simulink model "Fixed_SquadCopter_Closed_Loop_SMC"  (R2023a)
settings: Solver=ode4  StartTime=0.0  StopTime=20  FixedStep=0.01  RelTol=1e-3
undefined symbols (not defined in the file): sigbuilder_block
libraries: simulink_extras x23
settings Model: Creator=karee  LastModifiedBy=Nada Tamer
settings SolverCC: AlgebraicLoopSolver=TrustRegion
settings DataIOCC: ReturnWorkspaceOutputs=off
settings DebuggingCC: UnconnectedInputMsg=warning  UnconnectedOutputMsg=warning  UnconnectedLineMsg=warning  ArithmeticOperatorsInVariantConditions=warning
settings ModelReferenceCC: EnableRefExpFcnMdlSchedulingChecks=on
settings SFSimCC: SimUseLocalCustomCode=off  CustomCodeUndefinedFunction=UseInterfaceOnly
settings RTWCC: RTWUseLocalCustomCode=off

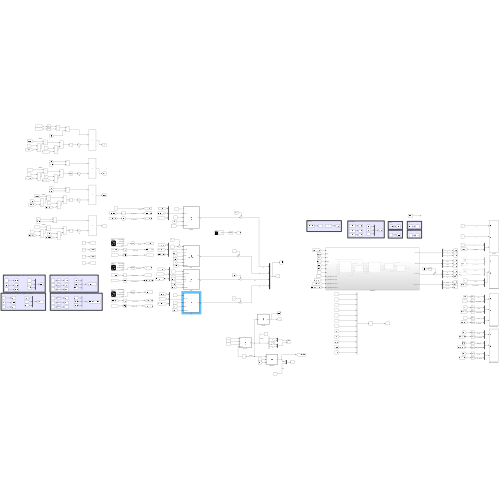
[thumbnail: Simulink's stored preview of the top-level diagram]
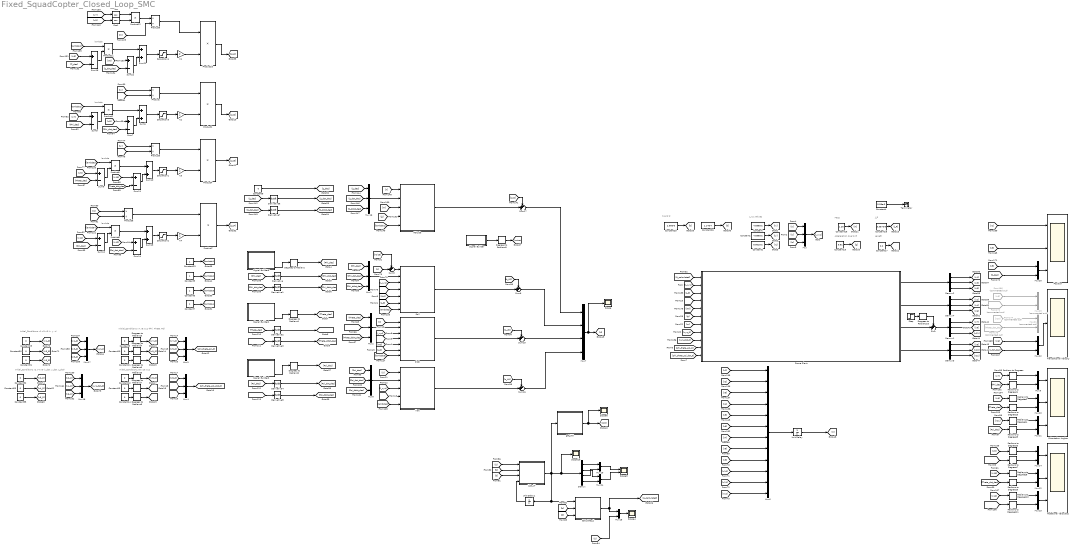
== system Fixed_SquadCopter_Closed_Loop_SMC ==
  note: b and d
  note: lambda
  note: Acceleration due to G
  note: I_xyz Values
  note: Mass
  note: Length
  note: J_R
  note: lambda
  note: lambda
  note: Initial_Conditions x7,x9,x11 (Phi, Theta, Psi)
  note: Initial_Conditions x8,x10,x12
  note: lambda
  note: Initial_Conditions x1,x3,x5 (x, y, z)
  note: Initial_Conditions x2,x4,x6 (x_dot, y_dot, z_dot)
  Attitude : MATLAB Function  TreatAsAtomicUnit=on
  Calculate_U : MATLAB Function  TreatAsAtomicUnit=on
  Constant : Constant  Value=4.856e-2
  Constant1 : Constant  Value=4.856e-2
  Constant{8..14,29..33,35} (13 alike) : Constant  Value=0
  Constant15 : Constant  Value=9.81
  Constant16 : Constant  Value=1.26
  Constant17 : Constant  Value=0.2
  Constant18 : Constant  Value=3.357e-5
  Constant2 : Constant  Value=8.801e-2
  Constant{5..7,23} (4 alike) : Constant
  Constant25 : Constant  Value=2.98e-6
  Constant26 : Constant  Value=1.14e-7
  Constant4 : Constant  Value=5.58e-3
  Cos : Trigonometry  Operator=cos
  Cos1 : Trigonometry  Operator=cos
  Degrees to Radians{,1..10} (11 alike) : simulink_extras/Transformations/Degrees to Radians
  Demux : Demux
  Demux{1..4} (4 alike) : Demux  Outputs=3
  Derivative{,1..7} (8 alike) : Derivative
  Drone Plant : Subsystem
  From166 : From  Commented=on  GotoTag=x8
  From172 : From  Commented=on  GotoTag=Phi_dot_des
  From173 : From  Commented=on  GotoTag=Theta_dot_des
  From174 : From  Commented=on  GotoTag=x10
  K{1..4} (4 alike) : Gain  Gain=2
  Mux{,1..4,8,16..18} (9 alike) : Mux  Inputs=3
  Mux{9..15,19..20,22,24} (11 alike) : Mux  Inputs=2
  Mux21 : Mux  Commented=on  Inputs=2
  Mux23 : Mux  Commented=on  Inputs=2
  Mux6 : Mux  Inputs=12
  Mux7 : Mux
  Orientation Angles : Scope  NumInputPorts=3
  Pitch : MATLAB Function  TreatAsAtomicUnit=on
  Position : Scope  NumInputPorts=3
  Product{,3,6,9} (4 alike) : Product  Inputs=*/
  Product{1..2,4..5,7..8,10..12} (9 alike) : Product  Inputs=**
  Radians to Degrees{,1..11} (12 alike) : simulink_extras/Transformations/Radians to Degrees
  Roll : MATLAB Function  TreatAsAtomicUnit=on
  Rotational Velocities : Scope  NumInputPorts=3
  Saturation{1..4} (4 alike) : Saturate  UpperLimit=1  LowerLimit=-1
  Scope{,4,6,10} (4 alike) : Scope
  Scope3 : Scope  NumInputPorts=2
  Signal Builder : Subsystem  Tag=STV Subsys  LoadFcn=sigbuilder_block('load');  StartFcn=sigbuilder_block('start');  StopFcn=sigbuilder_block('stop');  ClipboardFcn=sigbuilder_block('clipboard');  mask(Sigbuilder block){tuvar=[0:10]}
      mask help: Simulink:masks:SigbuilderBlock_MD
      mask init:
      | if ~strcmp(get_param(bdroot(gcbh),'SimulationStatus'),'stopped') tuvar = sigbuilder_block('maskInit'); end
      settings: CopyFcn=sigbuilder_block('copy');  DeleteFcn=sigbuilder_block('delete');  ModelCloseFcn=sigbuilder_block('modelClose');  PreSaveFcn=sigbuilder_block('preSave');  PauseFcn=sigbuilder_block('pause');  ContinueFcn=sigbuilder_block('continue');  NameChangeFcn=sigbuilder_block('namechange');  OpenFcn=sigbuilder_block('open',[437.25 153 550.5 359.25 ]);  CloseFcn=sigbuilder_block('close');
      mask Display: plot(0, 0, 100, 100,[2, 2, 32, 32, 2], [68, 8, 8, 68, 68],[32, 2], [38, 38], [32, 19, 2],[53, 60, 44], [32, 17, 17, 2],[16, 16, 31, 31]);txt = getActiveGroup(gcbh);text(2, 100, txt,'verticalAlignment', 'top');
  Signal Builder1 : Subsystem  Tag=STV Subsys  LoadFcn=sigbuilder_block('load');  StartFcn=sigbuilder_block('start');  StopFcn=sigbuilder_block('stop');  ClipboardFcn=sigbuilder_block('clipboard');  mask(Sigbuilder block){tuvar=[0:10]}
      mask help: Simulink:masks:SigbuilderBlock_MD
      mask init:
      | if ~strcmp(get_param(bdroot(gcbh),'SimulationStatus'),'stopped') tuvar = sigbuilder_block('maskInit'); end
      settings: CopyFcn=sigbuilder_block('copy');  DeleteFcn=sigbuilder_block('delete');  ModelCloseFcn=sigbuilder_block('modelClose');  PreSaveFcn=sigbuilder_block('preSave');  PauseFcn=sigbuilder_block('pause');  ContinueFcn=sigbuilder_block('continue');  NameChangeFcn=sigbuilder_block('namechange');  OpenFcn=sigbuilder_block('open',[0 30 1024.5 488.25 ]);  CloseFcn=sigbuilder_block('close');
      mask Display: plot(0, 0, 100, 100,[2, 2, 32, 32, 2], [68, 8, 8, 68, 68],[32, 2], [38, 38], [32, 19, 2],[53, 60, 44], [32, 17, 17, 2],[16, 16, 31, 31]);txt = getActiveGroup(gcbh);text(2, 100, txt,'verticalAlignment', 'top');
  Signal Builder2 : Subsystem  Tag=STV Subsys  LoadFcn=sigbuilder_block('load');  StartFcn=sigbuilder_block('start');  StopFcn=sigbuilder_block('stop');  ClipboardFcn=sigbuilder_block('clipboard');  mask(Sigbuilder block){tuvar=[0:10]}
      mask help: Simulink:masks:SigbuilderBlock_MD
      mask init:
      | if ~strcmp(get_param(bdroot(gcbh),'SimulationStatus'),'stopped') tuvar = sigbuilder_block('maskInit'); end
      settings: CopyFcn=sigbuilder_block('copy');  DeleteFcn=sigbuilder_block('delete');  ModelCloseFcn=sigbuilder_block('modelClose');  PreSaveFcn=sigbuilder_block('preSave');  PauseFcn=sigbuilder_block('pause');  ContinueFcn=sigbuilder_block('continue');  NameChangeFcn=sigbuilder_block('namechange');  OpenFcn=sigbuilder_block('open',[6 30 1012.5 447.75 ]);  CloseFcn=sigbuilder_block('close');
      mask Display: plot(0, 0, 100, 100,[2, 2, 32, 32, 2], [68, 8, 8, 68, 68],[32, 2], [38, 38], [32, 19, 2],[53, 60, 44], [32, 17, 17, 2],[16, 16, 31, 31]);txt = getActiveGroup(gcbh);text(2, 100, txt,'verticalAlignment', 'top');
  Signal Builder3 : Subsystem  Tag=STV Subsys  LoadFcn=sigbuilder_block('load');  StartFcn=sigbuilder_block('start');  StopFcn=sigbuilder_block('stop');  ClipboardFcn=sigbuilder_block('clipboard');  mask(Sigbuilder block){tuvar=[0:10]}
      mask help: Simulink:masks:SigbuilderBlock_MD
      mask init:
      | if ~strcmp(get_param(bdroot(gcbh),'SimulationStatus'),'stopped') tuvar = sigbuilder_block('maskInit'); end
      settings: CopyFcn=sigbuilder_block('copy');  DeleteFcn=sigbuilder_block('delete');  ModelCloseFcn=sigbuilder_block('modelClose');  PreSaveFcn=sigbuilder_block('preSave');  PauseFcn=sigbuilder_block('pause');  ContinueFcn=sigbuilder_block('continue');  NameChangeFcn=sigbuilder_block('namechange');  OpenFcn=sigbuilder_block('open',[6 30 1012.5 447.75 ]);  CloseFcn=sigbuilder_block('close');
      mask Display: plot(0, 0, 100, 100,[2, 2, 32, 32, 2], [68, 8, 8, 68, 68],[32, 2], [38, 38], [32, 19, 2],[53, 60, 44], [32, 17, 17, 2],[16, 16, 31, 31]);txt = getActiveGroup(gcbh);text(2, 100, txt,'verticalAlignment', 'top');
  Step : Step  Time=10  After=0  SampleTime=0
  Sum : Sum  Inputs=++|
  Sum{6,10,13,21} (4 alike) : Sum
  Sum{5,7,9,11..12,14,18,22} (8 alike) : Sum  Inputs=+-
  Sum{8,15..17} (4 alike) : Sum  Inputs=-+|
  Sum3 : Sum  Inputs=++|
  Terminator : Terminator
  Translational Velocity : Scope
  U_to_W : MATLAB Function  TreatAsAtomicUnit=on
  Unit Delay : UnitDelay  InitialCondition=[0;0;0;0;0;0;0;0;0;0;0;0]  SampleTime=0.01  HasFrameUpgradeWarning=on
  Unit Delay1 : UnitDelay  InitialCondition=[1018;1018;1018;1018]  SampleTime=0.01  HasFrameUpgradeWarning=on
  Yaw : MATLAB Function  TreatAsAtomicUnit=on
  get_Wd : MATLAB Function  TreatAsAtomicUnit=on
  wires:
  [Iz] -> Mux/3
  Constant1/1 -> [Iy]
  Constant2/1 -> [Iz]
  [Iy] -> Mux/2
  Constant/1 -> [Ix]
  Mux/1 -> [I_xyz]
  [Ix] -> Mux/1
  Constant15/1 -> [g]
  Constant16/1 -> [m]
  Constant17/1 -> [length]
  Constant18/1 -> [J_R]
  Constant25/1 -> [b]
  Constant26/1 -> [d]
  Demux1/3 -> [x11]  "psi"
  Demux1/2 -> [x9]  "theta"
  Demux3/1 -> [x8]  "phi_dot"
  Demux3/2 -> [x10]  "theta_dot"
  Demux3/3 -> [x12]  "psi_dot"
  [x8] -> Mux6/8
  [x10] -> Mux6/10
  [x12] -> Mux6/12
  Mux6/1 -> Unit Delay/1
  [I_xyz] -> Roll/3(I_xyz)
  [length] -> Roll/4(length)
  Mux7/1 -> Scope/1, [U]
  [U] -> U_to_W/1(U)
  [Wd] -> Roll/5(w_d)
  Mux1/1 -> Roll/2(PHI_des)
  Degrees to Radians/1 -> [Phi_des]  "Phi_des"
  [Phi_dot_des] -> Mux1/2
  [Phi_ddot_des] -> Mux1/3
  Mux2/1 -> Pitch/2(THETA_des)
  [X] -> Pitch/1(X)
  [I_xyz] -> Pitch/3(I_xyz)
  [length] -> Pitch/4(length)
  [Wd] -> Pitch/5(w_d)
  [I_xyz] -> Yaw/3(I_xyz)
  [X] -> Yaw/1(X)
  Mux8/1 -> Yaw/2(PSI_des)
  [length] -> Yaw/4(length)
  [x5] -> Mux6/5
  [x6] -> Mux6/6
  Unit Delay/1 -> [X]
  [J_R] -> Roll/6(J_r)
  [J_R] -> Pitch/6(J_r)
  [Ix] -> Product/1
  [length] -> Product/2
  Product/1 -> Product1/1
  [x7] -> Sum5/1
  [Phi_des] -> Mux1/1
  Derivative/1 -> [Phi_dot_des]  "Phi_dot_des"
  Derivative1/1 -> [Phi_ddot_des]  "Phi_ddot_des"
  [Phi_des] -> Sum5/2
  [lambda2] -> Product2/1
  Sum5/1 -> Product2/2
  Product2/1 -> Sum6/1
  [Phi_dot_des] -> Sum7/2
  [x8] -> Sum7/1
  Sum7/1 -> Sum6/2
  Sum6/1 -> Saturation3/1
  Saturation3/1 -> K2/1
  Roll/1(U2) -> Sum8/2  "U2"
  Sum8/1 -> Mux7/2  "U2"
  Derivative3/1 -> [Theta_ddot_des]  "Theta_ddot_des"
  Derivative2/1 -> [Theta_dot_des]  "Theta_dot_des"
  Degrees to Radians1/1 -> [Theta_des]  "Theta_des"
  [Theta_ddot_des] -> Mux2/3
  [Theta_des] -> Mux2/1
  [Theta_dot_des] -> Mux2/2
  Sum9/1 -> Product5/2
  [x10] -> Sum11/1
  Sum10/1 -> Saturation1/1
  Product3/1 -> Product4/1
  [length] -> Product3/2
  [x9] -> Sum9/1
  Sum11/1 -> Sum10/2
  [lambda3] -> Product5/1
  Saturation1/1 -> K3/1
  Product5/1 -> Sum10/1
  [Theta_des] -> Sum9/2
  [Theta_dot_des] -> Sum11/2
  [Iy] -> Product3/1
  Sum12/1 -> Product8/2
  [x12] -> Sum14/1
  Sum13/1 -> Saturation2/1
  Product6/1 -> Product7/1
  [length] -> Product6/2
  [x11] -> Sum12/1
  Sum14/1 -> Sum13/2
  [lambda4] -> Product8/1
  Saturation2/1 -> K4/1
  Product8/1 -> Sum13/1
  [Psi_des] -> Sum12/2
  [Psi_dot_des] -> Sum14/2
  [Iz] -> Product6/1
  Product1/1 -> [s_U2]
  Product4/1 -> [s_U3]
  Product7/1 -> [s_U4]
  Pitch/1(U3) -> Sum15/2  "U3"
  Yaw/1(U4) -> Sum16/2  "U4"
  Sum16/1 -> Mux7/4  "U4"
  Sum15/1 -> Mux7/3  "U3"
  [s_U2] -> Sum8/1
  [s_U3] -> Sum15/1
  [s_U4] -> Sum16/1
  Degrees to Radians2/1 -> [Psi_des]  "Psi_des"
  Derivative4/1 -> [Psi_dot_des]  "Psi_dot_des"
  Derivative5/1 -> [Psi_ddot_des]  "Psi_ddot_des"
  [Psi_des] -> Mux8/1
  [Psi_dot_des] -> Mux8/2
  [Psi_ddot_des] -> Mux8/3
  K4/1 -> Product7/2
  K3/1 -> Product4/2
  K2/1 -> Product1/2
  Mux9/1 -> Orientation Angles/1
  [x7] -> Radians to Degrees/1
  [Phi_des] -> Radians to Degrees1/1
  [Theta_des] -> Radians to Degrees3/1
  [x9] -> Radians to Degrees2/1
  Mux10/1 -> Orientation Angles/2
  Mux11/1 -> Orientation Angles/3
  [x11] -> Radians to Degrees4/1
  [Psi_des] -> Radians to Degrees5/1
  [Psi_dot_des] -> Radians to Degrees11/1
  [x12] -> Radians to Degrees10/1
  Mux13/1 -> Rotational Velocities/3
  Mux12/1 -> Rotational Velocities/2
  [x10] -> Radians to Degrees8/1
  [Theta_dot_des] -> Radians to Degrees9/1
  [Phi_dot_des] -> Radians to Degrees7/1
  [x8] -> Radians to Degrees6/1
  Mux14/1 -> Rotational Velocities/1
  Radians to Degrees/1 -> Mux9/1  "Phi"
  Radians to Degrees1/1 -> Mux9/2  "Phi_desired"
  Radians to Degrees2/1 -> Mux10/1  "Theta"
  Radians to Degrees3/1 -> Mux10/2  "Theta_desired"
  Radians to Degrees4/1 -> Mux11/1  "Psi"
  Radians to Degrees5/1 -> Mux11/2  "Psi_desired"
  Radians to Degrees7/1 -> Mux14/2  "Phi_dot_desired"
  Radians to Degrees6/1 -> Mux14/1  "Phi_dot"
  Radians to Degrees8/1 -> Mux12/1  "Theta_dot"
  Radians to Degrees9/1 -> Mux12/2  "Theta_dot_desired"
  Radians to Degrees10/1 -> Mux13/1  "Psi_dot"
  Radians to Degrees11/1 -> Mux13/2  "Psi_dot_desired"
  [Phi_des] -> Derivative/1
  [Phi_dot_des] -> Derivative1/1
  [Theta_dot_des] -> Derivative3/1
  [Theta_des] -> Derivative2/1
  [Psi_des] -> Derivative4/1
  [Theta_dot_des] -> Derivative5/1
  [d] -> U_to_W/3(d)
  [b] -> U_to_W/2(b)
  [b] -> Calculate_U/2(b)
  [d] -> Calculate_U/3(d)
  U_to_W/1(W) -> Scope10/1, Demux/1, get_Wd/1(W), Unit Delay1/1, Calculate_U/1(W)  "Omegas"
  Calculate_U/1(U) -> [U_calculated], Mux15/1  "Ucalc"
  [U] -> Mux15/2  "Uact"
  get_Wd/1(Wd) -> Scope6/1, [Wd]
  Constant5/1 -> [lambda2]
  Constant6/1 -> [lambda3]
  Constant7/1 -> [lambda4]
  [lambda2] -> Roll/7(lambda2)
  [lambda3] -> Pitch/7(lambda3)
  [lambda4] -> Yaw/5(lambda4)
  Constant14/1 -> Degrees to Radians8/1
  Degrees to Radians8/1 -> [x12_0]
  [x7_0] -> Mux3/1
  Degrees to Radians3/1 -> [x7_0]
  Degrees to Radians5/1 -> [x11_0]
  Mux3/1 -> [phi_theta_psi_0]
  Degrees to Radians4/1 -> [x9_0]
  [x9_0] -> Mux3/2
  [x12_0] -> Mux4/3
  Mux4/1 -> [phi_theta_psi_dot_0]
  Constant11/1 -> Degrees to Radians5/1
  Constant10/1 -> Degrees to Radians4/1
  [x10_0] -> Mux4/2
  [x8_0] -> Mux4/1
  Constant12/1 -> Degrees to Radians6/1
  Degrees to Radians7/1 -> [x10_0]
  Constant13/1 -> Degrees to Radians7/1
  Constant9/1 -> Degrees to Radians3/1
  Degrees to Radians6/1 -> [x8_0]
  [x11_0] -> Mux3/3
  [g] -> Attitude/4(g)
  Mux16/1 -> Attitude/2(Z_des)
  [lambda1] -> Attitude/5(lambda1)
  Constant8/1 -> [Z_des]  "Phi_des"
  [X] -> Attitude/1(X)
  Derivative6/1 -> [Z_dot_des]  "Phi_dot_des"
  [Z_des] -> Mux16/1
  [Z_dot_des] -> Derivative7/1
  Sum17/1 -> Mux7/1  "U1"
  [Z_dot_des] -> Mux16/2
  [s_U1] -> Sum17/1
  Derivative7/1 -> [Z_ddot_des]  "Phi_ddot_des"
  Attitude/1(U1) -> Sum17/2  "U1"
  [m] -> Attitude/3(m)
  [Z_des] -> Derivative6/1
  [Z_ddot_des] -> Mux16/3
  Product12/1 -> Product9/1
  Cos/1 -> Product12/1
  [m] -> Product9/2
  [x9] -> Cos1/1
  [x7] -> Cos/1
  [Z_des] -> Sum18/2
  Saturation4/1 -> K1/1
  [x6] -> Sum22/1
  [lambda1] -> Product11/1
  [Z_dot_des] -> Sum22/2
  Sum22/1 -> Sum21/2
  K1/1 -> Product10/2
  Product10/1 -> [s_U1]
  Sum18/1 -> Product11/2
  [x5] -> Sum18/1
  Product9/1 -> Product10/1
  Sum21/1 -> Saturation4/1
  Product11/1 -> Sum21/1
  Cos1/1 -> Product12/2
  [U_calculated] -> Drone Plant/1(u)
  Drone Plant/4("x8, x10, x12") -> Demux3/1
  [I_xyz] -> Drone Plant/2(I_xyz)
  [phi_theta_psi_dot_0] -> Drone Plant/11("Init_Conditions x8, x10, x12,")
  [xyz_dot_0] -> Drone Plant/9("Init_Conditions x2, x4, x6,")
  [J_R] -> Drone Plant/3(J_R)
  [xyz_0] -> Drone Plant/8("Init_Conditions x1, x3, x5")
  [phi_theta_psi_0] -> Drone Plant/10("Init_Conditions x7, x9, x11,")
  [g] -> Drone Plant/6(g)
  [length] -> Drone Plant/4(length)
  [m] -> Drone Plant/7(m)
  [Wd] -> Drone Plant/5(wd)
  Demux4/3 -> [x6]  "z_dot"
  Demux4/2 -> [x4]  "y_dot"
  Demux4/1 -> [x2]  "x_dot"
  Demux2/1 -> [x1]  "x"
  Demux2/2 -> [x3]  "y"
  Demux2/3 -> [x5]  "z"
  Drone Plant/2("x2, x4, x6") -> Demux4/1
  Drone Plant/1("x1, x3, x5") -> Demux2/1
  Constant33/1 -> [x4_0]
  [x5_0] -> Mux17/3
  Constant30/1 -> [x3_0]
  [x3_0] -> Mux17/2
  Mux17/1 -> [xyz_0]
  [x6_0] -> Mux18/3
  Constant35/1 -> [x6_0]
  [x4_0] -> Mux18/2
  [x1_0] -> Mux17/1
  Constant29/1 -> [x1_0]
  Constant31/1 -> [x5_0]
  [x2_0] -> Mux18/1
  Mux18/1 -> [xyz_dot_0]
  Constant32/1 -> [x2_0]
  [Z_dot_des] -> Mux22/2  "Z_dot_desired"
  [x6] -> Mux22/1  "Z_dot"
  From173/1 -> Mux21/2  "Theta_dot_desired"
  From174/1 -> Mux21/1  "Theta_dot"
  From166/1 -> Mux23/1  "Phi_dot"
  From172/1 -> Mux23/2  "Phi_dot_desired"
  [Z_des] -> Mux20/2  "Z_desired"
  [x5] -> Mux20/1  "Z"
  [x3] -> Position/2  "Y"
  [x1] -> Position/1  "X"
  Mux22/1 -> Translational Velocity/1
  Constant23/1 -> [lambda1]
  Demux1/1 -> [x7]  "phi"
  Mux20/1 -> Position/3
  [x4] -> Mux6/4
  [x3] -> Mux6/3
  [x2] -> Mux6/2
  [x1] -> Mux6/1
  Demux/1 -> Mux19/1  "w1"
  Mux19/1 -> Scope3/1
  Demux/3 -> Mux19/2  "w3"
  Mux24/1 -> Scope3/2
  Demux/2 -> Mux24/1  "w2"
  Demux/4 -> Mux24/2  "w4"
  Constant4/1 -> Terminator/1
  Mux15/1 -> Scope4/1
  Unit Delay1/1 -> U_to_W/4(W_old)
  Signal Builder1/4(Zero) -> Degrees to Radians1/1
  Signal Builder/1(Noise) -> Degrees to Radians9/1
  Degrees to Radians9/1 -> [noise]
  [x7] -> Mux6/7
  [x9] -> Mux6/9
  [x11] -> Mux6/11
  [noise] -> Sum3/1
  Sum3/1 -> Roll/1(X)
  [X] -> Sum3/2
  Sum/1 -> Demux1/1
  Drone Plant/3("x7, x9, x11") -> Sum/2
  Step/1 -> Degrees to Radians10/1
  Signal Builder3/4(Zero) -> Degrees to Radians/1
  Degrees to Radians10/1 -> Sum/1
  Signal Builder2/4(Zero) -> Degrees to Radians2/1

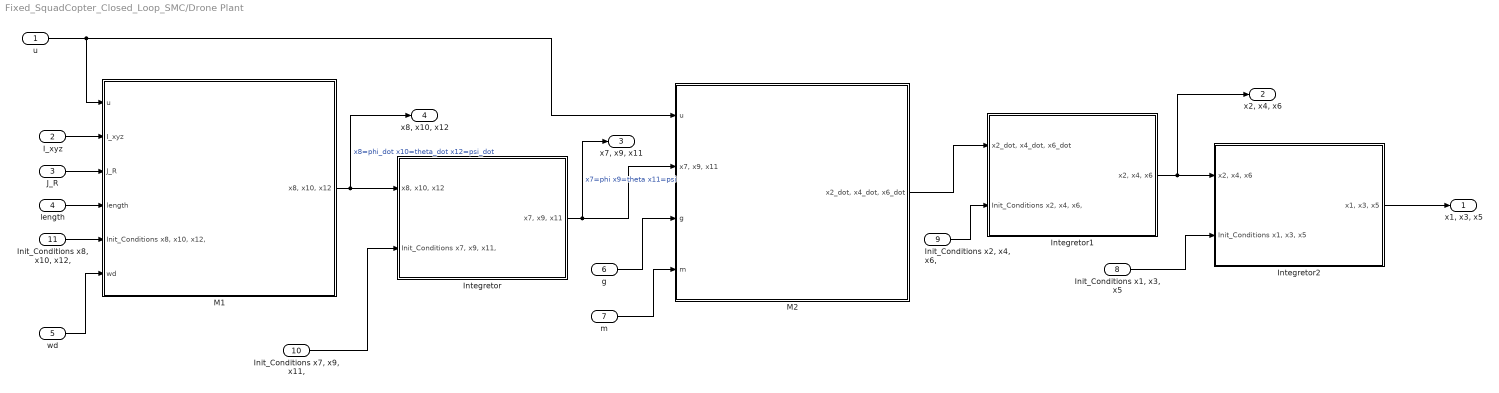
== system Fixed_SquadCopter_Closed_Loop_SMC/Drone Plant ==
  u : Inport
  I_xyz : Inport  Port=2
  J_R : Inport  Port=3
  length : Inport  Port=4
  wd : Inport  Port=5
  g : Inport  Port=6
  m : Inport  Port=7
  "Init_Conditions x1, x3, x5" : Inport  Port=8
  "Init_Conditions x2, x4, x6," : Inport  Port=9
  "Init_Conditions x7, x9, x11," : Inport  Port=10
  "Init_Conditions x8, x10, x12," : Inport  Port=11
  Integretor : Subsystem
  Integretor1 : Subsystem
  Integretor2 : Subsystem
  M1 : Subsystem
  M2 : Subsystem
  "x1, x3, x5" : Outport  VectorParamsAs1DForOutWhenUnconnected=off
  "x2, x4, x6" : Outport  Port=2  VectorParamsAs1DForOutWhenUnconnected=off
  "x7, x9, x11" : Outport  Port=3  VectorParamsAs1DForOutWhenUnconnected=off
  "x8, x10, x12" : Outport  Port=4  VectorParamsAs1DForOutWhenUnconnected=off
  wires:
  Integretor2/1("x1, x3, x5") -> "x1, x3, x5"/1
  Integretor1/1("x2, x4, x6") -> "x2, x4, x6"/1, Integretor2/1("x2, x4, x6")
  Integretor/1("x7, x9, x11") -> "x7, x9, x11"/1, M2/2("x7, x9, x11")  "x7=phi x9=theta x11=psi"
  u/1 -> M1/1(u), M2/1(u)
  m/1 -> M2/4(m)
  M1/1("x8, x10, x12") -> "x8, x10, x12"/1, Integretor/1("x8, x10, x12")  "x8=phi_dot x10=theta_dot x12=psi_dot"
  "Init_Conditions x7, x9, x11,"/1 -> Integretor/2("Init_Conditions x7, x9, x11,")
  g/1 -> M2/3(g)
  "Init_Conditions x2, x4, x6,"/1 -> Integretor1/2("Init_Conditions x2, x4, x6,")
  "Init_Conditions x1, x3, x5"/1 -> Integretor2/2("Init_Conditions x1, x3, x5")
  "Init_Conditions x8, x10, x12,"/1 -> M1/5("Init_Conditions x8, x10, x12,")
  length/1 -> M1/4(length)
  M2/1("x2_dot, x4_dot, x6_dot") -> Integretor1/1("x2_dot, x4_dot, x6_dot")
  wd/1 -> M1/6(wd)
  J_R/1 -> M1/3(J_R)
  I_xyz/1 -> M1/2(I_xyz)

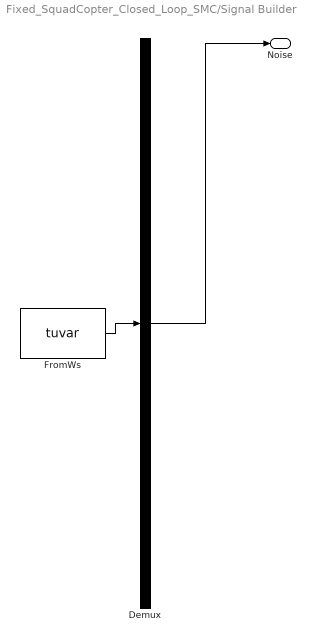
== system Fixed_SquadCopter_Closed_Loop_SMC/Signal Builder ==
  Demux : Demux  Tag=STV Demux  Outputs=1
      settings: DisplayOption=none
  FromWs : FromWorkspace  Tag=STV FromWs  VariableName=tuvar
      SigBuilderData=|
      | common.afterFinalStr = 'Extrapolate'
      | common.sampleTime = 0
      | dataSet.timeRange = [0 20]
      | dataSet.name = 'Group 1'
      | sbobj.Groups.Name = 'Group 1'
      | sbobj.Groups.Signals.Name = 'Noise'
      | sbobj.Groups.Signals.XData = [0 1 2 3 4 5 6 7 8 9 10 11 12 13 14 15 16 17 18 19 20]
      | sbobj.Groups.Signals.YData = [0.942376933302 0.0937254906669 -1.12231172153 0.306157818568 -1.17233486755 -0.960966563538 -0.653735016358 -1.229393649 -0.270965129963 -0.899950067343 -0.285686137602 -0.462421544354 -0.40978521474 -0.503538984132 1.23329711264 0.610305217574 0.0590721550527 -1.46694673043 -1.6258032664 -1.96475241539 2.60519575087]
      | sbobj.Groups.TimeRange = [0 20]
  Noise : Outport  Tag=STV Outport  VectorParamsAs1DForOutWhenUnconnected=off
  wires:
  Demux/1 -> Noise/1
  FromWs/1 -> Demux/1

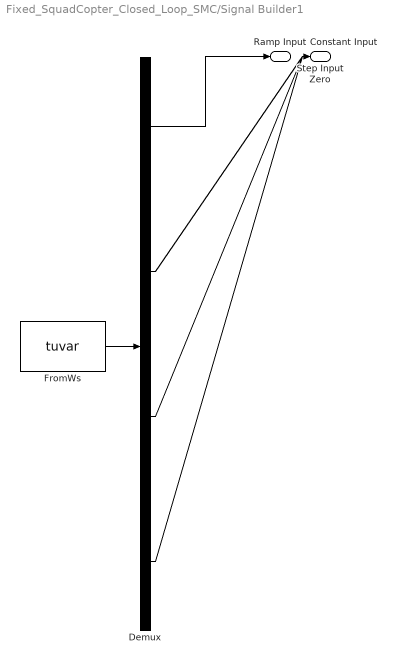
== system Fixed_SquadCopter_Closed_Loop_SMC/Signal Builder1 ==
  Demux : Demux  Tag=STV Demux
      settings: DisplayOption=none
  FromWs : FromWorkspace  Tag=STV FromWs  VariableName=tuvar
      SigBuilderData=|
      | common.afterFinalStr = 'Extrapolate'
      | common.sampleTime = 0
      | dataSet.timeRange = [0 20]
      | dataSet.name = 'Group 1'
      | sbobj.Groups.Name = 'Group 1'
      | sbobj.Groups.Signals(1).Name = 'Ramp Input'
      | sbobj.Groups.Signals(1).XData = [0 20]
      | sbobj.Groups.Signals(1).YData = [0 15]
      | sbobj.Groups.Signals(2).Name = 'Step Input'
      | sbobj.Groups.Signals(2).XData = [0 5 5 10 10 15 15 20]
      | sbobj.Groups.Signals(2).YData = [0 0 15 15 10 10 0 0]
      | sbobj.Groups.Signals(3).Name = 'Constant Input'
      | sbobj.Groups.Signals(3).XData = [0 20]
      | sbobj.Groups.Signals(3).YData = [10 10]
      | sbobj.Groups.Signals(4).Name = 'Zero'
      | sbobj.Groups.Signals(4).XData = [0 20]
      | sbobj.Groups.Signals(4).YData = [0 0]
      | sbobj.Groups.TimeRange = [0 20]
  Ramp Input : Outport  Tag=STV Outport  VectorParamsAs1DForOutWhenUnconnected=off
  Step Input : Outport  Tag=STV Outport  Port=2  VectorParamsAs1DForOutWhenUnconnected=off
  Constant Input : Outport  Tag=STV Outport  Port=3  VectorParamsAs1DForOutWhenUnconnected=off
  Zero : Outport  Tag=STV Outport  Port=4  VectorParamsAs1DForOutWhenUnconnected=off
  wires:
  Demux/3 -> Constant Input/1
  Demux/2 -> Step Input/1
  FromWs/1 -> Demux/1
  Demux/1 -> Ramp Input/1
  Demux/4 -> Zero/1

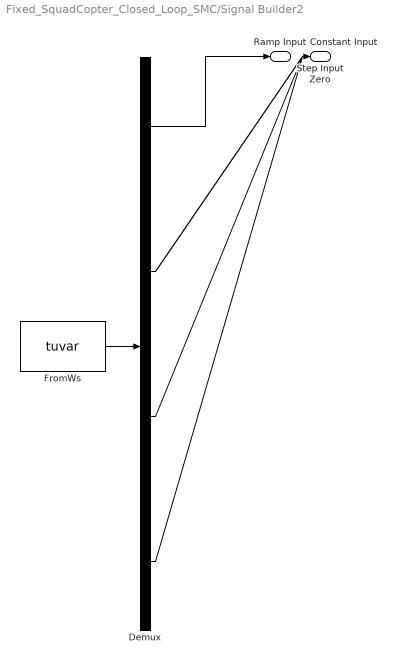
== system Fixed_SquadCopter_Closed_Loop_SMC/Signal Builder2 ==
  Demux : Demux  Tag=STV Demux
      settings: DisplayOption=none
  FromWs : FromWorkspace  Tag=STV FromWs  VariableName=tuvar
      SigBuilderData=|
      | common.afterFinalStr = 'Extrapolate'
      | common.sampleTime = 0
      | dataSet.timeRange = [0 20]
      | dataSet.name = 'Group 1'
      | sbobj.Groups.Name = 'Group 1'
      | sbobj.Groups.Signals(1).Name = 'Ramp Input'
      | sbobj.Groups.Signals(1).XData = [0 20]
      | sbobj.Groups.Signals(1).YData = [0 360]
      | sbobj.Groups.Signals(2).Name = 'Step Input'
      | sbobj.Groups.Signals(2).XData = [0 5 5 10 10 15 15 20]
      | sbobj.Groups.Signals(2).YData = [0 0 90 90 45 45 0 0]
      | sbobj.Groups.Signals(3).Name = 'Constant Input'
      | sbobj.Groups.Signals(3).XData = [0 20]
      | sbobj.Groups.Signals(3).YData = [180 180]
      | sbobj.Groups.Signals(4).Name = 'Zero'
      | sbobj.Groups.Signals(4).XData = [0 20]
      | sbobj.Groups.Signals(4).YData = [0 0]
      | sbobj.Groups.TimeRange = [0 20]
  Ramp Input : Outport  Tag=STV Outport  VectorParamsAs1DForOutWhenUnconnected=off
  Step Input : Outport  Tag=STV Outport  Port=2  VectorParamsAs1DForOutWhenUnconnected=off
  Constant Input : Outport  Tag=STV Outport  Port=3  VectorParamsAs1DForOutWhenUnconnected=off
  Zero : Outport  Tag=STV Outport  Port=4  VectorParamsAs1DForOutWhenUnconnected=off
  wires:
  Demux/1 -> Ramp Input/1
  FromWs/1 -> Demux/1
  Demux/2 -> Step Input/1
  Demux/3 -> Constant Input/1
  Demux/4 -> Zero/1

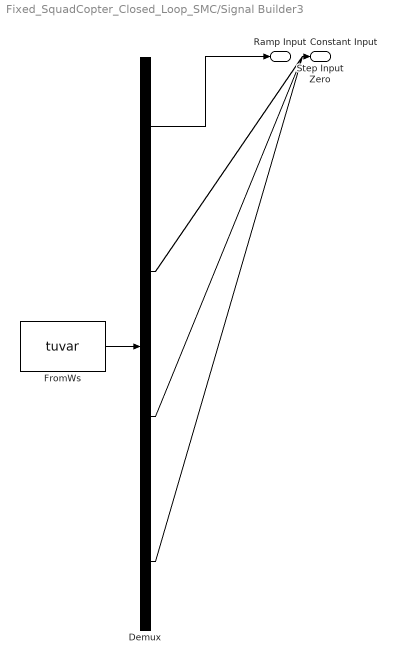
== system Fixed_SquadCopter_Closed_Loop_SMC/Signal Builder3 ==
  Demux : Demux  Tag=STV Demux
      settings: DisplayOption=none
  FromWs : FromWorkspace  Tag=STV FromWs  VariableName=tuvar
      SigBuilderData=|
      | common.afterFinalStr = 'Extrapolate'
      | common.sampleTime = 0
      | dataSet.timeRange = [0 20]
      | dataSet.name = 'Group 1'
      | sbobj.Groups.Name = 'Group 1'
      | sbobj.Groups.Signals(1).Name = 'Ramp Input'
      | sbobj.Groups.Signals(1).XData = [0 20]
      | sbobj.Groups.Signals(1).YData = [0 20]
      | sbobj.Groups.Signals(2).Name = 'Step Input'
      | sbobj.Groups.Signals(2).XData = [0 5 5 10 10 15 15 20]
      | sbobj.Groups.Signals(2).YData = [0 0 25 25 10 10 0 0]
      | sbobj.Groups.Signals(3).Name = 'Constant Input'
      | sbobj.Groups.Signals(3).XData = [0 20]
      | sbobj.Groups.Signals(3).YData = [20 20]
      | sbobj.Groups.Signals(4).Name = 'Zero'
      | sbobj.Groups.Signals(4).XData = [0 20]
      | sbobj.Groups.Signals(4).YData = [0 0]
      | sbobj.Groups.TimeRange = [0 20]
  Ramp Input : Outport  Tag=STV Outport  VectorParamsAs1DForOutWhenUnconnected=off
  Step Input : Outport  Tag=STV Outport  Port=2  VectorParamsAs1DForOutWhenUnconnected=off
  Constant Input : Outport  Tag=STV Outport  Port=3  VectorParamsAs1DForOutWhenUnconnected=off
  Zero : Outport  Tag=STV Outport  Port=4  VectorParamsAs1DForOutWhenUnconnected=off
  wires:
  Demux/4 -> Zero/1
  Demux/3 -> Constant Input/1
  Demux/2 -> Step Input/1
  FromWs/1 -> Demux/1
  Demux/1 -> Ramp Input/1

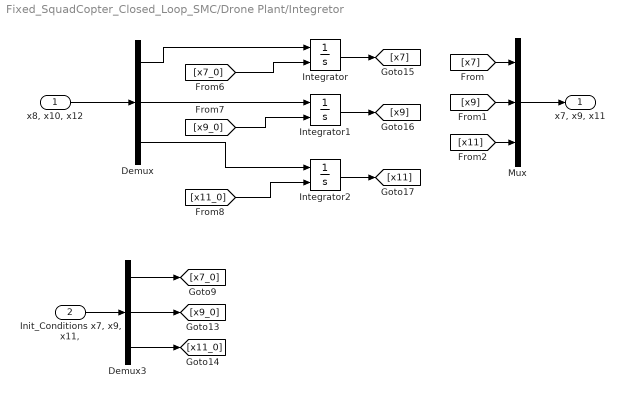
== system Fixed_SquadCopter_Closed_Loop_SMC/Drone Plant/Integretor ==
  "x8, x10, x12" : Inport
  "Init_Conditions x7, x9, x11," : Inport  Port=2
  Demux : Demux  Outputs=3
  Demux3 : Demux  Outputs=3
  Integrator : Integrator  InitialConditionSource=external
  Integrator1 : Integrator  InitialConditionSource=external
  Integrator2 : Integrator  InitialConditionSource=external
  Mux : Mux  Inputs=3
  "x7, x9, x11" : Outport  VectorParamsAs1DForOutWhenUnconnected=off
  wires:
  [x7] -> Mux/1
  [x11] -> Mux/3
  Demux3/3 -> [x11_0]
  Integrator2/1 -> [x11]
  [x11_0] -> Integrator2/2
  [x9] -> Mux/2
  "Init_Conditions x7, x9, x11,"/1 -> Demux3/1
  [x7_0] -> Integrator/2
  Mux/1 -> "x7, x9, x11"/1
  [x9_0] -> Integrator1/2
  Integrator/1 -> [x7]
  Demux/1 -> Integrator/1
  Integrator1/1 -> [x9]
  "x8, x10, x12"/1 -> Demux/1
  Demux/2 -> Integrator1/1
  Demux3/2 -> [x9_0]
  Demux3/1 -> [x7_0]
  Demux/3 -> Integrator2/1

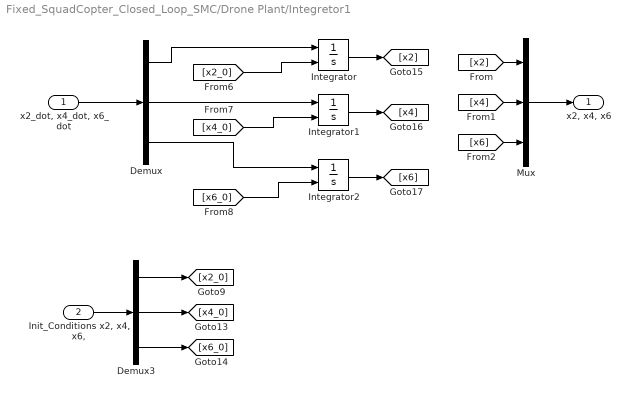
== system Fixed_SquadCopter_Closed_Loop_SMC/Drone Plant/Integretor1 ==
  "x2_dot, x4_dot, x6_dot" : Inport
  "Init_Conditions x2, x4, x6," : Inport  Port=2
  Demux : Demux  Outputs=3
  Demux3 : Demux  Outputs=3
  Integrator : Integrator  InitialConditionSource=external
  Integrator1 : Integrator  InitialConditionSource=external
  Integrator2 : Integrator  InitialConditionSource=external
  Mux : Mux  Inputs=3
  "x2, x4, x6" : Outport  VectorParamsAs1DForOutWhenUnconnected=off
  wires:
  Demux/3 -> Integrator2/1
  Demux3/1 -> [x2_0]
  Demux3/2 -> [x4_0]
  Demux/2 -> Integrator1/1
  "x2_dot, x4_dot, x6_dot"/1 -> Demux/1
  Integrator1/1 -> [x4]
  Demux/1 -> Integrator/1
  Integrator/1 -> [x2]
  [x4_0] -> Integrator1/2
  Mux/1 -> "x2, x4, x6"/1
  [x2_0] -> Integrator/2
  "Init_Conditions x2, x4, x6,"/1 -> Demux3/1
  [x4] -> Mux/2
  [x6_0] -> Integrator2/2
  Integrator2/1 -> [x6]
  Demux3/3 -> [x6_0]
  [x6] -> Mux/3
  [x2] -> Mux/1

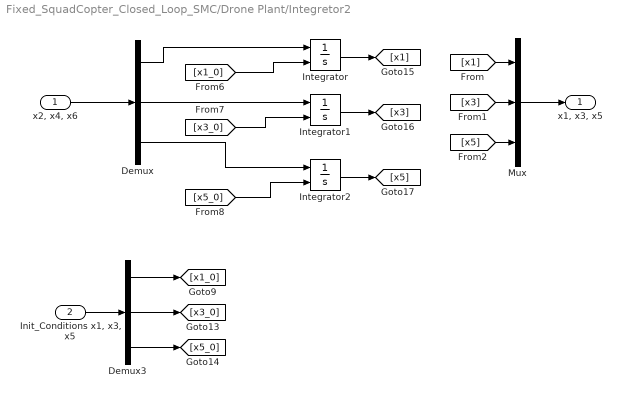
== system Fixed_SquadCopter_Closed_Loop_SMC/Drone Plant/Integretor2 ==
  "x2, x4, x6" : Inport
  "Init_Conditions x1, x3, x5" : Inport  Port=2
  Demux : Demux  Outputs=3
  Demux3 : Demux  Outputs=3
  Integrator : Integrator  InitialConditionSource=external
  Integrator1 : Integrator  InitialConditionSource=external
  Integrator2 : Integrator  InitialConditionSource=external
  Mux : Mux  Inputs=3
  "x1, x3, x5" : Outport  VectorParamsAs1DForOutWhenUnconnected=off
  wires:
  [x1] -> Mux/1
  [x5] -> Mux/3
  Demux3/3 -> [x5_0]
  Integrator2/1 -> [x5]
  [x5_0] -> Integrator2/2
  [x3] -> Mux/2
  "Init_Conditions x1, x3, x5"/1 -> Demux3/1
  [x1_0] -> Integrator/2
  Mux/1 -> "x1, x3, x5"/1
  [x3_0] -> Integrator1/2
  Integrator/1 -> [x1]
  Demux/1 -> Integrator/1
  Integrator1/1 -> [x3]
  "x2, x4, x6"/1 -> Demux/1
  Demux/2 -> Integrator1/1
  Demux3/2 -> [x3_0]
  Demux3/1 -> [x1_0]
  Demux/3 -> Integrator2/1

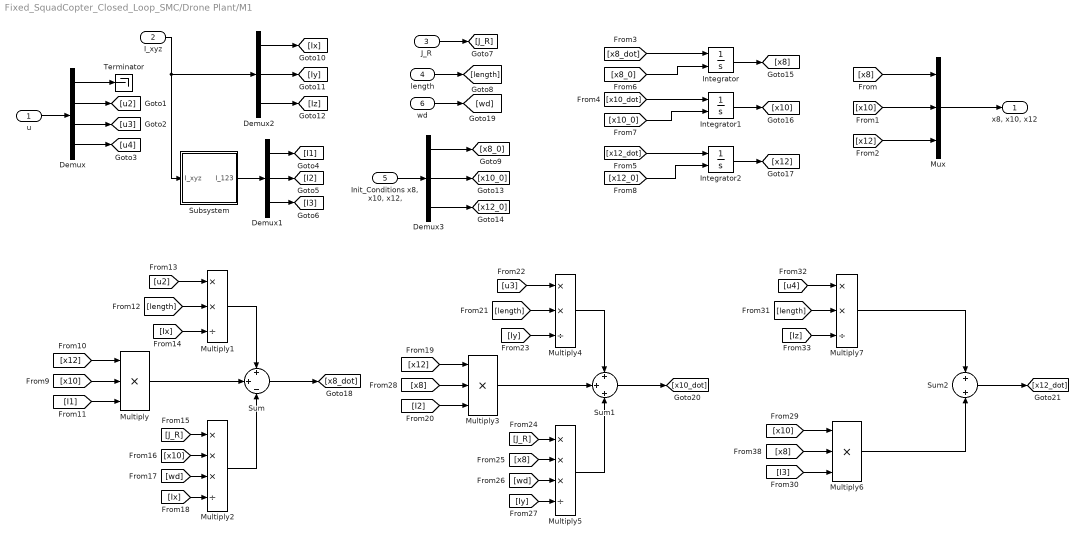
== system Fixed_SquadCopter_Closed_Loop_SMC/Drone Plant/M1 ==
  u : Inport
  I_xyz : Inport  Port=2
  J_R : Inport  Port=3
  length : Inport  Port=4
  "Init_Conditions x8, x10, x12," : Inport  Port=5
  wd : Inport  Port=6
  Demux : Demux
  Demux1 : Demux  Outputs=3
  Demux2 : Demux  Outputs=3
  Demux3 : Demux  Outputs=3
  Integrator : Integrator  InitialConditionSource=external
  Integrator1 : Integrator  InitialConditionSource=external
  Integrator2 : Integrator  InitialConditionSource=external
  Multiply : Product  Inputs=3
  Multiply1 : Product  Inputs=**/
  Multiply2 : Product  Inputs=***/
  Multiply3 : Product  Inputs=3
  Multiply4 : Product  Inputs=**/
  Multiply5 : Product  Inputs=***/
  Multiply6 : Product  Inputs=3
  Multiply7 : Product  Inputs=**/
  Mux : Mux  Inputs=3
  Subsystem : Subsystem
  Sum : Sum  Inputs=+|+|-
  Sum1 : Sum  Inputs=+|+|+
  Sum2 : Sum  Inputs=+|+
  Terminator : Terminator
  "x8, x10, x12" : Outport  VectorParamsAs1DForOutWhenUnconnected=off
  wires:
  u/1 -> Demux/1
  Demux/1 -> Terminator/1
  Demux/2 -> [u2]
  Demux/3 -> [u3]
  Demux/4 -> [u4]
  Demux2/2 -> [Iy]
  Demux2/3 -> [Iz]
  Demux2/1 -> [Ix]
  I_xyz/1 -> Demux2/1, Subsystem/1(I_xyz)
  Subsystem/1(I_123) -> Demux1/1
  Demux1/1 -> [I1]
  Demux1/2 -> [I2]
  Demux1/3 -> [I3]
  J_R/1 -> [J_R]
  length/1 -> [length]
  "Init_Conditions x8, x10, x12,"/1 -> Demux3/1
  Demux3/1 -> [x8_0]
  Demux3/3 -> [x12_0]
  Demux3/2 -> [x10_0]
  [x10] -> Mux/2
  [x8] -> Mux/1
  [x12] -> Mux/3
  Mux/1 -> "x8, x10, x12"/1
  [x12_dot] -> Integrator2/1
  [x8_dot] -> Integrator/1
  [x10_dot] -> Integrator1/1
  [x8_0] -> Integrator/2
  [x10_0] -> Integrator1/2
  [x12_0] -> Integrator2/2
  Integrator/1 -> [x8]
  Integrator1/1 -> [x10]
  Integrator2/1 -> [x12]
  Sum/1 -> [x8_dot]
  Multiply/1 -> Sum/2
  [x12] -> Multiply/1
  [x10] -> Multiply/2
  [I1] -> Multiply/3
  wd/1 -> [wd]
  [length] -> Multiply1/2
  [u2] -> Multiply1/1
  [Ix] -> Multiply1/3
  Multiply1/1 -> Sum/1
  [J_R] -> Multiply2/1
  [x10] -> Multiply2/2
  [wd] -> Multiply2/3
  [Ix] -> Multiply2/4
  Multiply2/1 -> Sum/3
  Multiply5/1 -> Sum1/3
  [Iy] -> Multiply5/4
  [wd] -> Multiply5/3
  [x8] -> Multiply5/2
  [J_R] -> Multiply5/1
  Multiply4/1 -> Sum1/1
  [Iy] -> Multiply4/3
  [u3] -> Multiply4/1
  [length] -> Multiply4/2
  [I2] -> Multiply3/3
  [x8] -> Multiply3/2
  [x12] -> Multiply3/1
  Multiply3/1 -> Sum1/2
  Sum1/1 -> [x10_dot]
  Sum2/1 -> [x12_dot]
  Multiply6/1 -> Sum2/2
  [x10] -> Multiply6/1
  [x8] -> Multiply6/2
  [I3] -> Multiply6/3
  [length] -> Multiply7/2
  [u4] -> Multiply7/1
  [Iz] -> Multiply7/3
  Multiply7/1 -> Sum2/1

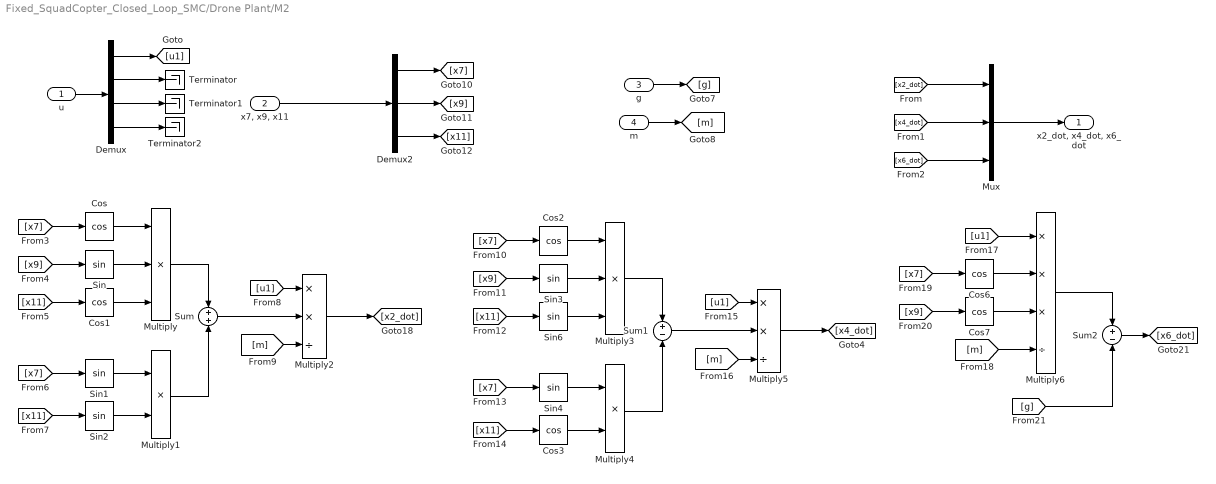
== system Fixed_SquadCopter_Closed_Loop_SMC/Drone Plant/M2 ==
  u : Inport
  "x7, x9, x11" : Inport  Port=2
  g : Inport  Port=3
  m : Inport  Port=4
  Cos{,1..3,6..7} (6 alike) : Trigonometry  Operator=cos
  Demux : Demux
  Demux2 : Demux  Outputs=3
  Multiply : Product  Inputs=3
  Multiply1 : Product
  Multiply2 : Product  Inputs=**/
  Multiply3 : Product  Inputs=3
  Multiply4 : Product
  Multiply5 : Product  Inputs=**/
  Multiply6 : Product  Inputs=***/
  Mux : Mux  Inputs=3
  Sin{,1..4,6} (6 alike) : Trigonometry
  Sum : Sum  Inputs=+|+
  Sum1 : Sum  Inputs=+|-
  Sum2 : Sum  Inputs=+|-
  Terminator : Terminator
  Terminator1 : Terminator
  Terminator2 : Terminator
  "x2_dot, x4_dot, x6_dot" : Outport  VectorParamsAs1DForOutWhenUnconnected=off
  wires:
  Mux/1 -> "x2_dot, x4_dot, x6_dot"/1
  [x6_dot] -> Mux/3
  [x2_dot] -> Mux/1
  [x4_dot] -> Mux/2
  m/1 -> [m]
  g/1 -> [g]
  Demux/4 -> Terminator2/1
  Demux/3 -> Terminator1/1
  Demux/2 -> Terminator/1
  Demux/1 -> [u1]
  u/1 -> Demux/1
  "x7, x9, x11"/1 -> Demux2/1
  Demux2/1 -> [x7]
  Demux2/3 -> [x11]
  Demux2/2 -> [x9]
  Multiply/1 -> Sum/1
  Multiply1/1 -> Sum/2
  Sum/1 -> Multiply2/2
  Multiply2/1 -> [x2_dot]
  Sin/1 -> Multiply/2
  Cos/1 -> Multiply/1
  Cos1/1 -> Multiply/3
  [x7] -> Cos/1
  [x9] -> Sin/1
  [x11] -> Cos1/1
  Sin1/1 -> Multiply1/1
  Sin2/1 -> Multiply1/2
  [x7] -> Sin1/1
  [x11] -> Sin2/1
  [u1] -> Multiply2/1
  [m] -> Multiply2/3
  [m] -> Multiply5/3
  [u1] -> Multiply5/1
  [x11] -> Cos3/1
  [x7] -> Sin4/1
  Cos3/1 -> Multiply4/2
  Sin4/1 -> Multiply4/1
  [x11] -> Sin6/1
  [x9] -> Sin3/1
  [x7] -> Cos2/1
  Sin6/1 -> Multiply3/3
  Cos2/1 -> Multiply3/1
  Sin3/1 -> Multiply3/2
  Multiply5/1 -> [x4_dot]
  Sum1/1 -> Multiply5/2
  Multiply4/1 -> Sum1/2
  Multiply3/1 -> Sum1/1
  [x9] -> Cos7/1
  Cos7/1 -> Multiply6/3
  Cos6/1 -> Multiply6/2
  [x7] -> Cos6/1
  [u1] -> Multiply6/1
  [m] -> Multiply6/4
  Multiply6/1 -> Sum2/1
  [g] -> Sum2/2
  Sum2/1 -> [x6_dot]

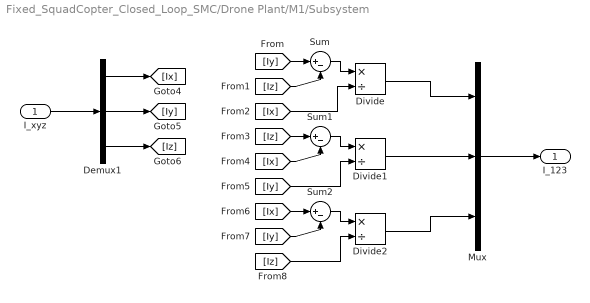
== system Fixed_SquadCopter_Closed_Loop_SMC/Drone Plant/M1/Subsystem ==
  I_xyz : Inport
  Demux1 : Demux  Outputs=3
  Divide : Product  Inputs=*/
  Divide1 : Product  Inputs=*/
  Divide2 : Product  Inputs=*/
  Mux : Mux  Inputs=3
  Sum : Sum  Inputs=|+-
  Sum1 : Sum  Inputs=|+-
  Sum2 : Sum  Inputs=|+-
  I_123 : Outport  VectorParamsAs1DForOutWhenUnconnected=off
  wires:
  [Iy] -> Sum2/2
  Divide2/1 -> Mux/3
  [Iy] -> Sum/1
  Sum/1 -> Divide/1
  I_xyz/1 -> Demux1/1
  Sum2/1 -> Divide2/1
  [Ix] -> Sum2/1
  [Iz] -> Divide2/2
  Demux1/3 -> [Iz]
  [Ix] -> Sum1/2
  Demux1/1 -> [Ix]
  [Ix] -> Divide/2
  [Iz] -> Sum/2
  Divide/1 -> Mux/1
  Sum1/1 -> Divide1/1
  Divide1/1 -> Mux/2
  [Iz] -> Sum1/1
  [Iy] -> Divide1/2
  Demux1/2 -> [Iy]
  Mux/1 -> I_123/1

== matlab function Fixed_SquadCopter_Closed_Loop_SMC/Roll ==
  data: X input; U2 output; PHI_des input; I_xyz input; length input; w_d input; J_r input; lambda2 input
function U2 = Roll_Control(X,PHI_des,I_xyz,length,w_d,J_r,lambda2)
lambda=lambda2;
% k1=2;
% k2=2;
k=2;

Ix=I_xyz(1);
Iy=I_xyz(2);
Iz=I_xyz(3);

b1=length/Ix;

a1=(Iy-Iz)/Ix;

Phi=X(7);
Phi_dot=X(8);

Theta_dot=X(10);
Psi_dot=X(12);

Phi_des=PHI_des(1);
Phi_dot_des=PHI_des(2); 
Phi_ddot_des=PHI_des(3);

s=(-Phi_dot_des+Phi_dot)+lambda*(-Phi_des+Phi);
% s_dot=-k1*sign(s)-k2*s;

f=Psi_dot*Theta_dot*a1-(J_r/Ix)*Theta_dot*w_d;
% U2 = (1/b1)*(-s_dot-a1*Theta_dot*Psi_dot+Phi_ddot_des+lambda*(Phi_dot_des-Phi_dot));
U2 = (1/b1)*(-f+Phi_ddot_des+lambda*(Phi_dot_des-Phi_dot));

== matlab function Fixed_SquadCopter_Closed_Loop_SMC/Pitch ==
  data: X input; U3 output; THETA_des input; I_xyz input; length input; w_d input; J_r input; lambda3 input
function U3 = Pitch_Control(X,THETA_des,I_xyz,length,w_d,J_r,lambda3)
lambda=lambda3;
% k1=2;
% k2=2;
k=2;

Ix=I_xyz(1);
Iy=I_xyz(2);
Iz=I_xyz(3);

b1=length/Iy;

a2=(Iz-Ix)/Iy;

Phi=X(7);
Phi_dot=X(8);

Theta=X(9);
Theta_dot=X(10);

Psi=X(11);
Psi_dot=X(12);

Theta_des=THETA_des(1);
Theta_dot_des=THETA_des(2);
Theta_ddot_des=THETA_des(3);

s=(Theta_dot_des-Theta_dot)+lambda*(Theta_des-Theta);
% s_dot=-k1*sign(s)-k2*s;

f=Psi_dot*Phi_dot*a2+(J_r/Iy)*Phi_dot*w_d;
% U2 = (1/b1)*(-s_dot-a1*Theta_dot*Psi_dot+Phi_ddot_des+lambda*(Phi_dot_des-Phi_dot));
U3 = (1/b1)*(-f+Theta_ddot_des+lambda*(Theta_dot_des-Theta_dot));

== matlab function Fixed_SquadCopter_Closed_Loop_SMC/Calculate_U ==
  data: W input; U output; b input; d input
function U = fcn(W,b,d)
W1=W(1);
W2=W(2);
W3=W(3);
W4=W(4);
U1=b*(W4^2+W2^2+W3^2+W1^2);
U2=b*(W4^2-W2^2);
U3=b*(W3^2-W1^2);
U4=d*(W4^2+W2^2-W3^2-W1^2);

U=[U1;U2;U3;U4];
end

== matlab function Fixed_SquadCopter_Closed_Loop_SMC/get_Wd ==
  data: W input; Wd output
function Wd = fcn(W)
W1=W(1);
W2=W(2);
W3=W(3);
W4=W(4);
Wd=W4+W2-W3-W1;


end

== matlab function Fixed_SquadCopter_Closed_Loop_SMC/U_to_W ==
  data: U input; W output; b input; d input; W_old input
function W = fcn(U,b,d,W_old)
u1=U(1);
u2=U(2);
u3=U(3);
u4=U(4);

if (d*u1-2*d*u3-b*u4)/(4*d*b)>0
    w1=sqrt(((d*u1-2*d*u3-b*u4)/(4*d*b)));
else
    w1=W_old(1);
end

if ((d*u1-2*d*u2+b*u4)/(4*d*b))>0
    w2=sqrt(((d*u1-2*d*u2+b*u4)/(4*d*b)));
else
    w2=W_old(2);
end

if ((d*u1+2*d*u3-b*u4)/(4*d*b))>0
    w3=sqrt(((d*u1+2*d*u3-b*u4)/(4*d*b)));
else
    w3=W_old(3);
end

if ((d*u1+2*d*u2+b*u4)/(4*d*b))>0
    w4=sqrt(((d*u1+2*d*u2+b*u4)/(4*d*b)));
else
    w4=W_old(4);
end


W=[w1;w2;w3;w4];

== matlab function Fixed_SquadCopter_Closed_Loop_SMC/Yaw ==
  data: X input; U4 output; PSI_des input; I_xyz input; length input; lambda4 input
function U4 = Yaw_Control(X,PSI_des,I_xyz,length,lambda4)
lambda=lambda4;
% k1=2;
% k2=2;
k=2;

Ix=I_xyz(1);
Iy=I_xyz(2);
Iz=I_xyz(3);

b1=length/Iz;

a3=(Ix-Iy)/Iz;

Phi=X(7);
Phi_dot=X(8);

Theta=X(9);
Theta_dot=X(10);

Psi=X(11);
Psi_dot=X(12);

Psi_des=PSI_des(1);
Psi_dot_des=PSI_des(2);
Psi_ddot_des=PSI_des(3);

s=(Psi_dot_des-Psi_dot)+lambda*(Psi_des-Psi);
% s_dot=-k1*sign(s)-k2*s;

f=Theta_dot*Phi_dot*a3;
% U2 = (1/b1)*(-s_dot-a1*Theta_dot*Psi_dot+Phi_ddot_des+lambda*(Phi_dot_des-Phi_dot));
U4 = (1/b1)*(-f+Psi_ddot_des+lambda*(Psi_dot_des-Psi_dot));

== matlab function Fixed_SquadCopter_Closed_Loop_SMC/Attitude ==
  data: X input; U1 output; Z_des input; m input; g input; lambda1 input
function U1 = Attitude_Control(X,Z_des,m,g,lambda1)
lambda=lambda1;

z=X(5);
z_dot=X(6);

Phi=X(7);
Theta=X(9);

z_des=Z_des(1);
z_dot_des=Z_des(2); 
z_ddot_des=Z_des(3);


s=(-z_dot_des+z_dot)+lambda*(-z_des+z);
% s_dot=-k1*sign(s)-k2*s;

f=-g;
U1 = (m/(cos(Phi)*cos(Theta)))*(-f+z_ddot_des+lambda*(z_dot_des-z_dot));
